simulink model "Pderivativecontrol"  (R2021a)
settings: Solver=VariableStepAuto  StartTime=0.0  StopTime=3  RelTol=1e-3
values from neighbouring files (symbols this model uses):
  C = 2500*10^-6    (= 0.0025)    [parametrosRs.m]
  epsilon = 0.1    [parametrosRs.m]
  k2 = 1000    [parametrosRs.m]
  k3 = 3000    [parametrosRs.m]
  L = 10*10^-3    (= 0.01)    [parametrosRs.m]
  R = 0.1    [parametrosRs.m]
  w = 60    [parametrosRs.m]
  x2d = 0    [parametrosRs.m]
  x3d = 48    [parametrosRs.m]
undefined symbols (not defined in the file or in its folder): E_m
libraries: spsIGBTDiodeLib x6, spsCurrentMeasurementLib x4, spsSeriesRLCBranchLib x4, spsACVoltageSourceLib x3, eeTransforms x2, spsVoltageMeasurementLib x2, spsDCVoltageSourceLib x1, spsGroundLib x1, spsSVPWMGenerator2LevelLib x1, spsVariableResistorLib x1, spspowerguiLib x1
settings Model: Creator=CIO  LastModifiedBy=LAPONE

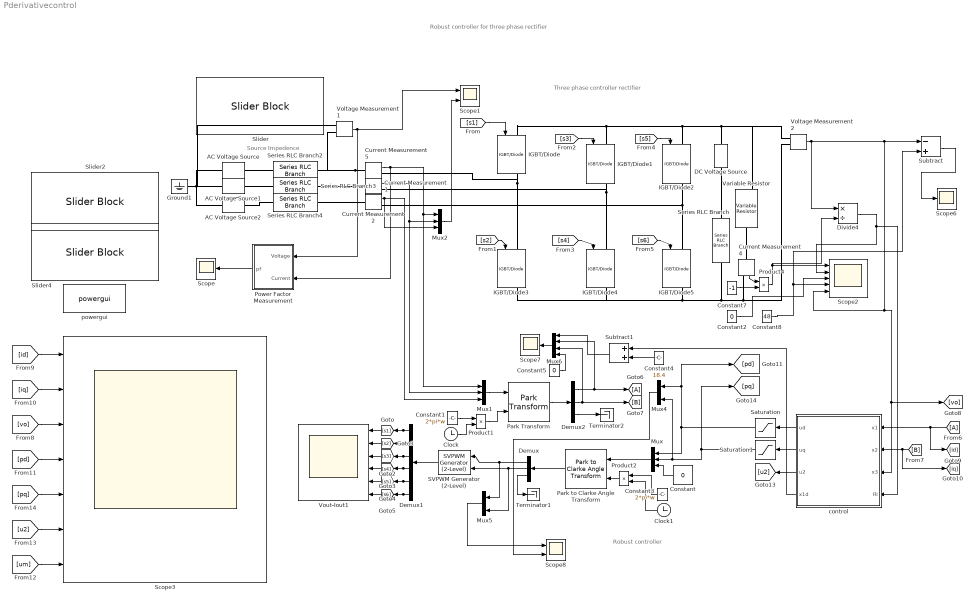
== system Pderivativecontrol ==
  note: Robust controller
  note: Source Impedence
  note: Three phase controller rectifier
  note: Robust controller for three phase rectifier
  AC Voltage Source : spsACVoltageSourceLib/AC Voltage Source  Amplitude=E_m  Phase=0  Frequency=w  SampleTime=0  Measurements=None  BusType=swing  Pref=10e3  Qref=0  Qmin=-inf  Qmax=+inf
  AC Voltage Source1 : spsACVoltageSourceLib/AC Voltage Source  Amplitude=E_m  Phase=240  Frequency=w  SampleTime=0  Measurements=None  BusType=swing  Pref=10e3  Qref=0  Qmin=-inf  Qmax=+inf
  AC Voltage Source2 : spsACVoltageSourceLib/AC Voltage Source  Amplitude=E_m  Phase=120  Frequency=w  SampleTime=0  Measurements=None  BusType=swing  Pref=10e3  Qref=0  Qmin=-inf  Qmax=+inf
  Clock : Clock
  Clock1 : Clock
  Constant : Constant  Value=0
  Constant1 : Constant  Value=2*pi*w
  Constant2 : Constant  Value=0
  Constant3 : Constant  Value=2*pi*w
  Constant4 : Constant  Value=18.4
  Constant5 : Constant  Value=0
  Constant7 : Constant  Value=-1
  Constant8 : Constant  Value=48
  Current Measurement{1..2,4..5} (4 alike) : spsCurrentMeasurementLib/Current Measurement  PhasorSimulation=off  OutputType=Magnitude  PSBequivalent=0
  DC Voltage Source : spsDCVoltageSourceLib/DC Voltage Source  Amplitude=0  Measurements=None
  Demux : Demux  Outputs=3
  Demux1 : Demux  Outputs=6
  Demux2 : Demux  Outputs=3
  Divide4 : Product  Inputs=*/
  Ground1 : spsGroundLib/Ground  LConnTagsString=a
  IGBT/Diode{,1..5} (6 alike) : spsIGBTDiodeLib/IGBT//Diode  Ron=1e-3  Rs=1e5  Cs=inf  Measurements=on
  Mux : Mux  Inputs=3
  Mux1 : Mux  Inputs=3
  Mux2 : Mux  Inputs=3
  Mux4 : Mux  Inputs=2
  Mux5 : Mux  Inputs=2
  Mux6 : Mux
  Park Transform : eeTransforms/Park Transform  AxisAlignment=D-axis  PowerInvariant=off
  Park to Clarke Angle Transform : eeTransforms/Park to Clarke Angle Transform  AxisAlignment=D-axis
      settings: SourceProductBaseCode=PS
  Power Factor Measurement : Subsystem
  Product1 : Product
  Product2 : Product
  Product4 : Product
  SVPWM Generator (2-Level) : spsSVPWMGenerator2LevelLib/SVPWM Generator (2-Level)  InputType=alpha-beta components  SwitchingPattern=Pattern #1  Fc=2500  ParUref=[0.8 -30 50]  Ts=0
      settings: SourceProductBaseCode=PS
  Saturation : Saturate  UpperLimit=50  LowerLimit=-50
  Saturation1 : Saturate  UpperLimit=25  LowerLimit=-25
  Scope : Scope
  Scope1 : Scope  NumInputPorts=2
  Scope2 : Scope  NumInputPorts=5
  Scope3 : Scope  NumInputPorts=7
  Scope6 : Scope
  Scope7 : Scope
  Scope8 : Scope  NumInputPorts=2
  Series RLC Branch : spsSeriesRLCBranchLib/Series RLC Branch  LConnTagsString=__new0  RConnTagsString=__new0  BranchType=C  Resistance=5  Inductance=1e-3  SetiL0=off  InitialCurrent=0  Capacitance=C  Setx0=off  InitialVoltage=0  Measurements=None
  Series RLC Branch2 : spsSeriesRLCBranchLib/Series RLC Branch  LConnTagsString=__new0  RConnTagsString=__new0  BranchType=RL  Resistance=R  Inductance=L  SetiL0=off  InitialCurrent=0  Capacitance=200e-6  Setx0=off  InitialVoltage=0  Measurements=Branch voltage and current
  Series RLC Branch3 : spsSeriesRLCBranchLib/Series RLC Branch  LConnTagsString=__new0  RConnTagsString=__new0  BranchType=RL  Resistance=R  Inductance=L  SetiL0=off  InitialCurrent=0  Capacitance=200e-6  Setx0=off  InitialVoltage=0  Measurements=Branch voltage and current
  Series RLC Branch4 : spsSeriesRLCBranchLib/Series RLC Branch  LConnTagsString=__new0  RConnTagsString=__new0  BranchType=RL  Resistance=R  Inductance=L  SetiL0=off  InitialCurrent=0  Capacitance=200e-6  Setx0=off  InitialVoltage=0  Measurements=Branch voltage and current
  Slider : SliderBlock  ScaleMin=10  ScaleMax=50
  Slider2 : SliderBlock  ScaleMax=5
  Slider4 : SliderBlock  ScaleMax=5
  Subtract : Sum  Inputs=-+
  Subtract1 : Sum
  Terminator1 : Terminator
  Terminator2 : Terminator
  Variable Resistor : spsVariableResistorLib/Variable Resistor  Rabsmin=17.38461538461539
      settings: SourceProductBaseCode=PS
  Voltage Measurement1 : spsVoltageMeasurementLib/Voltage Measurement  PhasorSimulation=off  OutputType=Magnitude  PSBequivalent=0
  Voltage Measurement2 : spsVoltageMeasurementLib/Voltage Measurement  PhasorSimulation=off  OutputType=Magnitude  PSBequivalent=0
  Vout-Iout1 : Scope  NumInputPorts=6
  control : MATLAB Function  TreatAsAtomicUnit=on
  powergui : spspowerguiLib/powergui  Priority=1  SimulationMode=Discrete  SampleTime=1e-6  frequency=60  Iterations=50  frequencyindice=0  Pbase=100e6  ErrMax=1e-4  UnitsV=kV  UnitsW=MW  buscounter=0  FunctionMessages=off  echomessages=off  EnableUseOfTLC=off  CurrentSourceSwitches=off  DisableSnubberDevices=off  DisableRonSwitches=off  DisableVfSwitches=off  DisplayEquations=off  AutomaticDiscreteSolvers=off  SolverType=Tustin/Backward Euler (TBE)  Interpol=off  ExternalGateDelay=off  methode=off  Ts=0  x0status=blocks  SPID=off  SwTol=0  HookPort=off  NonlinearTolerance=0  nMaxIteration=15  ContinueOnMaxIteration=off  RestoreLinks=warning  ResistiveCurrentMeasurement=off  Frange=[0:2:500]  Ylog=off  Xlog=on  ShowGrid=off  save=off  variable=ZData  structure=0  ZoomFFT=on  StartTime=0.0  cycles=1  DisplayStyle=1  fundamental=60  FreqAxis=off  MaxFrequency=1000  frequencyindicesteady=1  RmsSteady=1  display=off
  wires:
  [pq] -> Scope3/5
  [id] -> Scope3/1
  [u2] -> Scope3/6
  [vo] -> Scope3/3
  [um] -> Scope3/7
  [pd] -> Scope3/4
  [iq] -> Scope3/2
  Power Factor Measurement/1(pf) -> Scope/1
  Saturation/1 -> Mux/1, Mux4/1, [pd]
  Constant/1 -> Mux/3
  [B] -> [iq], control/2(x2)
  Mux1/1 -> Park Transform/1
  Demux1/5 -> Vout-Iout1/5, [s5]
  Voltage Measurement1/1 -> Power Factor Measurement/1(Voltage), Scope1/1
  Current Measurement1/1 -> Mux2/2, Mux1/2
  Demux1/1 -> Vout-Iout1/1, [s1]
  [s3] -> IGBT/Diode1/1
  Current Measurement5/1 -> Power Factor Measurement/2(Current), Mux2/1, Mux1/1
  Mux4/1 -> Scope8/2
  control/1(ud) -> Saturation/1
  Product4/1 -> Divide4/2, Scope2/1
  Constant1/1 -> Product1/1
  Current Measurement2/1 -> Mux2/3, Mux1/3
  [s2] -> IGBT/Diode3/1
  Product1/1 -> Park Transform/2
  Constant8/1 -> Subtract/2, Scope2/4
  Divide4/1 -> control/4(Rl), Scope2/2
  Demux2/3 -> Terminator2/1
  Product2/1 -> Park to Clarke Angle Transform/2
  Clock/1 -> Product1/2
  Clock1/1 -> Product2/2
  Constant4/1 -> Subtract1/2
  Park to Clarke Angle Transform/1 -> Demux/1
  Constant7/1 -> Product4/2
  Subtract1/1 -> Mux6/1
  Demux/3 -> Terminator1/1
  Saturation1/1 -> [pq], Mux4/2, Mux/2
  [s5] -> IGBT/Diode2/1
  Demux1/3 -> Vout-Iout1/3, [s3]
  Demux1/6 -> Vout-Iout1/6, [s6]
  Demux/2 -> Mux5/2, SVPWM Generator (2-Level)/2
  Demux1/4 -> Vout-Iout1/4, [s4]
  Mux6/1 -> Scope7/1
  Voltage Measurement2/1 -> Divide4/1, Scope2/5, [vo], control/3(x3), Subtract/1
  Mux/1 -> Park to Clarke Angle Transform/1
  [s4] -> IGBT/Diode4/1
  Demux1/2 -> Vout-Iout1/2, [s2]
  Park Transform/1 -> Demux2/1
  Constant2/1 -> Scope2/3
  SVPWM Generator (2-Level)/1 -> Demux1/1
  Current Measurement4/1 -> Product4/1
  [A] -> [id], control/1(x1)
  Subtract/1 -> Scope6/1
  Mux2/1 -> Scope1/2
  Constant3/1 -> Product2/1
  [s1] -> IGBT/Diode/1
  Demux2/1 -> [A], Mux6/2
  Mux5/1 -> Scope8/1
  Demux/1 -> Mux5/1, SVPWM Generator (2-Level)/1
  [s6] -> IGBT/Diode5/1
  control/2(uq) -> Saturation1/1
  Demux2/2 -> Mux6/3, [B]
  control/3(u2) -> [u2]
  control/4(x1d) -> Subtract1/1
  Constant5/1 -> Mux6/4
  connections:
  IGBT/Diode1/LConn1 -- IGBT/Diode/LConn1 -- IGBT/Diode2/LConn1 -- Variable Resistor/LConn1 -- Voltage Measurement2/LConn1 -- DC Voltage Source/RConn1
  AC Voltage Source1/RConn1 -- Ground1/LConn1 -- AC Voltage Source2/RConn1 -- Voltage Measurement1/LConn1 -- AC Voltage Source/RConn1
  Current Measurement2/RConn1 -- IGBT/Diode2/RConn1 -- IGBT/Diode5/LConn1
  Current Measurement5/LConn1 -- Series RLC Branch2/RConn1 -- Voltage Measurement1/LConn2
  Current Measurement1/RConn1 -- IGBT/Diode1/RConn1 -- IGBT/Diode4/LConn1
  Current Measurement4/RConn1 -- Voltage Measurement2/LConn2 -- Series RLC Branch/RConn1 -- IGBT/Diode4/RConn1 -- IGBT/Diode3/RConn1 -- IGBT/Diode5/RConn1
  IGBT/Diode/RConn1 -- IGBT/Diode3/LConn1 -- Current Measurement5/RConn1
  Series RLC Branch2/LConn1 -- AC Voltage Source/LConn1
  Series RLC Branch4/LConn1 -- AC Voltage Source2/LConn1
  Series RLC Branch3/RConn1 -- Current Measurement1/LConn1
  Series RLC Branch3/LConn1 -- AC Voltage Source1/LConn1
  Series RLC Branch4/RConn1 -- Current Measurement2/LConn1
  Variable Resistor/RConn1 -- Current Measurement4/LConn1
  Series RLC Branch/LConn1 -- DC Voltage Source/LConn1

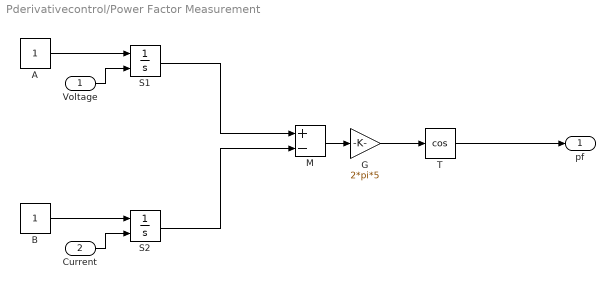
== system Pderivativecontrol/Power Factor Measurement ==
  Voltage : Inport
  Current : Inport  Port=2
  A : Constant
  B : Constant
  G : Gain  Gain=2*pi*5
  M : Sum  Inputs=+-
  S1 : Integrator  ExternalReset=falling
  S2 : Integrator  ExternalReset=falling
  T : Trigonometry  Operator=cos
  pf : Outport
  wires:
  A/1 -> S1/1
  B/1 -> S2/1
  S1/1 -> M/1
  S2/1 -> M/2
  Voltage/1 -> S1/2
  Current/1 -> S2/2
  M/1 -> G/1
  G/1 -> T/1
  T/1 -> pf/1

== matlab function Pderivativecontrol/control ==
  data: x1 input; ud output; x2 input; x3 input; uq output; E_m parameter; C parameter; L parameter; w parameter; R parameter; x3d parameter; x2d parameter; k3 parameter; k2 parameter; epsilon parameter; u2 output; x1d output; Rl input
function [ud , uq,u2,x1d] = fcn(x1, x2, x3, E_m, C, L, w, R, x3d, x2d, k3, k2, epsilon, Rl)


x1d_1 = (E_m/(2*R)) + (sqrt((E_m)^2 - (8*R*x3d^2)/(3*Rl)))/(2*R);
x1d_2 = (E_m/(2*R)) - (sqrt((E_m)^2 - (8*R*x3d^2)/(3*Rl)))/(2*R);
x1d = x1d_2;

%errors
e1 = x1 - x1d;      e2 = x2 - x2d;      e3 = x3 - x3d;  

%controls
%para evitar singularidades agregamos el termino epsilon donde corresponda
uq = (2*L/(x3 + epsilon)) * ( -(R/L)*(e2 + x2d) + w*(e1 + x1d) + k2*sqrt(abs(e2))*sign(e2) );

u2 = -(3/(4*C))*(e2 + x2d)*uq + (1/(Rl*C)) * (e3 + x3d) - k3*sqrt(abs(e3))*sign(e3);

ud =  ((4*C)/3) * u2/(x1 + epsilon) ;
